simulink model "baseon_xr_iter"  (R2017b)
settings: Solver=VariableStepAuto  StartTime=0.0  StopTime=45  RelTol=1e-3
PreLoadFcn:
  | init.m;
libraries: simulink x1
settings Model: Creator=Administrator  LastModifiedBy=Administrator
settings SolverCC: ZeroCrossAlgorithm=Adaptive  AlgebraicLoopSolver=LineSearch
settings DebuggingCC: MaxConsecutiveZCsMsg=none

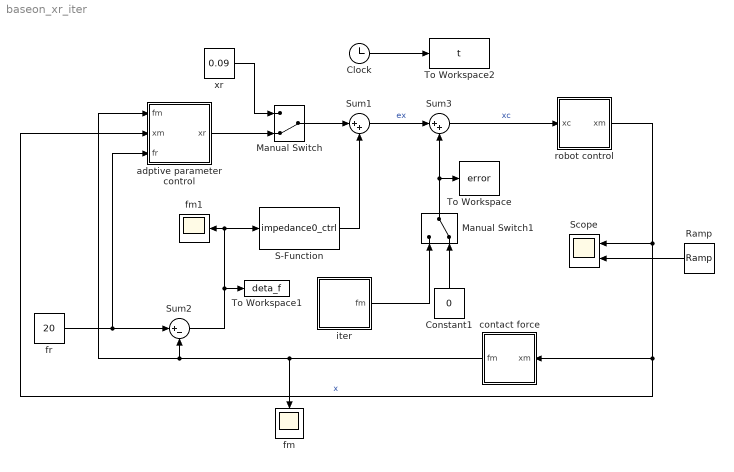
== system baseon_xr_iter ==
  Clock : Clock
  Constant1 : Constant  Value=0
  Manual Switch : ManualSwitch  CurrentSetting=0
  Manual Switch1 : ManualSwitch  CurrentSetting=0
  Ramp : simulink/Sources/Ramp  slope=1  start=0  X0=0
  S-Function : S-Function  FunctionName=impedance0_ctrl  SFunctionDeploymentMode=off  EnableBusSupport=off
  Scope : Scope  NumInputPorts=2
  Sum1 : Sum  Inputs=|++
  Sum2 : Sum  Inputs=|+-
  Sum3 : Sum  Inputs=|++
  To Workspace : ToWorkspace  VariableName=error  SampleTime=-1
      settings: Save2DSignal=2-D array (concatenate along first dimension)
  To Workspace1 : ToWorkspace  VariableName=deta_f  SampleTime=-1
      settings: Save2DSignal=2-D array (concatenate along first dimension)
  To Workspace2 : ToWorkspace  VariableName=t  SampleTime=-1
  adptive parameter control : Subsystem
  contact force : Subsystem
  fm : Scope
  fm1 : Scope
  fr : Constant  Value=20
  iter : Subsystem
  robot control : Subsystem
  xr : Constant  Value=0.09
  wires:
  adptive parameter control/1(xr) -> Manual Switch/2
  xr/1 -> Manual Switch/1
  Manual Switch/1 -> Sum1/1
  fr/1 -> adptive parameter control/3(fr), Sum2/1
  Sum1/1 -> Sum3/1  "ex"
  Manual Switch1/1 -> To Workspace/1, Sum3/2
  Constant1/1 -> Manual Switch1/2
  Sum3/1 -> robot control/1(xc)  "xc"
  robot control/1("xm ") -> adptive parameter control/2(xm), contact force/1(xm), Scope/1  "x"
  contact force/1("fm ") -> adptive parameter control/1(fm), Sum2/2, fm/1
  Ramp/1 -> Scope/2
  S-Function/1 -> Sum1/2
  Sum2/1 -> fm1/1, S-Function/1, To Workspace1/1
  iter/1("fm ") -> Manual Switch1/1
  Clock/1 -> To Workspace2/1

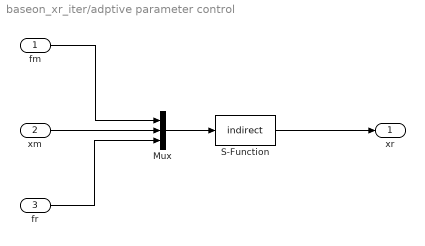
== system baseon_xr_iter/adptive parameter control ==
  fm : Inport
  xm : Inport  Port=2
  fr : Inport  Port=3
  Mux : Mux  Inputs=3
  S-Function : S-Function  FunctionName=indirect  SFunctionDeploymentMode=off  EnableBusSupport=off
  xr : Outport
  wires:
  fm/1 -> Mux/1
  xm/1 -> Mux/2
  Mux/1 -> S-Function/1
  S-Function/1 -> xr/1
  fr/1 -> Mux/3

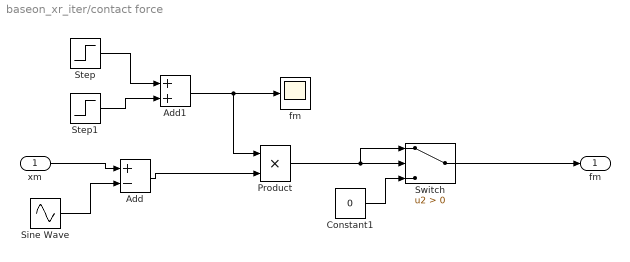
== system baseon_xr_iter/contact force ==
  xm : Inport
  Add : Sum  Inputs=+-
  Add1 : Sum
  Constant1 : Constant  Value=0
  Product : Product
  Sine Wave : Sin  Amplitude=0.01  SampleTime=0
  Step : Step  Time=15  Before=1500  After=2500  SampleTime=0
  Step1 : Step  Time=30  After=1500  SampleTime=0
  Switch : Switch  Criteria=u2 > Threshold
  fm : Scope
  "fm " : Outport
  wires:
  Add1/1 -> Product/1, fm/1
  xm/1 -> Add/1
  Add/1 -> Product/2
  Product/1 -> Switch/1, Switch/2
  Constant1/1 -> Switch/3
  Step/1 -> Add1/1
  Step1/1 -> Add1/2
  Switch/1 -> "fm "/1
  Sine Wave/1 -> Add/2

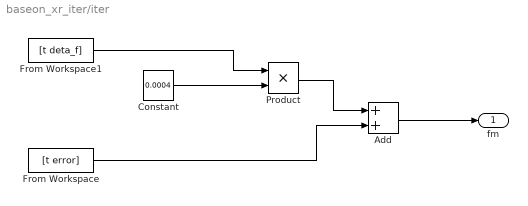
== system baseon_xr_iter/iter ==
  Add : Sum
  Constant : Constant  Value=0.0004
  From Workspace : FromWorkspace  VariableName=[t error]  SampleTime=0
  From Workspace1 : FromWorkspace  VariableName=[t deta_f]  SampleTime=0
  Product : Product
  "fm " : Outport
  wires:
  Constant/1 -> Product/2
  Product/1 -> Add/1
  From Workspace/1 -> Add/2
  Add/1 -> "fm "/1
  From Workspace1/1 -> Product/1

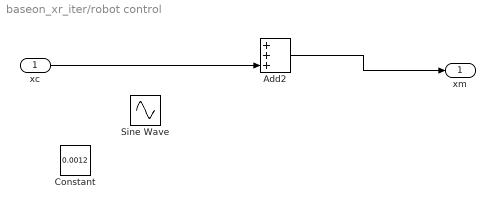
== system baseon_xr_iter/robot control ==
  xc : Inport
  Add2 : Sum  Inputs=+++
  Constant : Constant  Value=0.0012
  Sine Wave : Sin  Amplitude=0.001  Frequency=0.22  SampleTime=0.01
  "xm " : Outport
  wires:
  xc/1 -> Add2/3
  Add2/1 -> "xm "/1
